simulink model "katy_sym"  (R2016a)
settings: Solver=ode4  StartTime=0.0  StopTime=30  FixedStep=0.001  RelTol=1e-3
values from neighbouring files (symbols this model uses):
  A = [0 1 ... (first row only)    [por_model_obiekt_osX.m]    (also in wykresy.m)
  Ao = [0 1 ... (first row only)    [wykresy.m]
  B = [0; k/omega0^2]    [por_model_obiekt_osX.m]    (also in wykresy.m)
  Bo = [0; k1/omega01^2]    [wykresy.m]
  C = [1 0]    [por_model_obiekt_osX.m]    (also in wykresy.m)
  Co = [1 0]    [wykresy.m]
  D = 0    [por_model_obiekt_osX.m]    (also in wykresy.m)
  Do = 0    [wykresy.m]
  X0 = [0 0]    [por_model_obiekt_osX.m]    (also in wykresy.m = [0.2738 0])
settings Model: Creator=Maciek  LastModifiedBy=Maciek

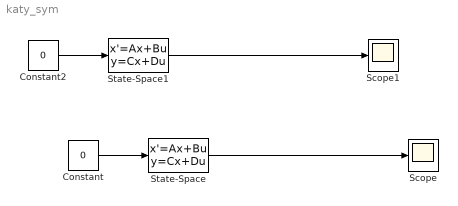
== system katy_sym ==
  Constant : Constant  Value=0
  Constant2 : Constant  Value=0
  Scope : Scope
  Scope1 : Scope
  State-Space : StateSpace  A=A  B=B  C=C  D=D  X0=X0
  State-Space1 : StateSpace  A=Ao  B=Bo  C=Co  D=Do  X0=X0
  wires:
  Constant/1 -> State-Space/1
  State-Space/1 -> Scope/1
  Constant2/1 -> State-Space1/1
  State-Space1/1 -> Scope1/1
